simulink model "angle_lut_stage4_harness"  (R2024b)
settings: Solver=VariableStepAuto  StartTime=0.0  StopTime=10.0  RelTol=1e-3
model workspace (MAT data in the model file):
  B = 0.008
  BW_I = 5000
  BW_speed = 20
  J = 5.5e-06
  Ld = 6.1e-05
  Lq = 6.1e-05
  Rs = 0.09
  T_ident = 5e-05
  Ts = 5e-06
  Vdc = 24
  adc_current_bits = 12
  adc_current_gain = 1
  adc_current_lsb_A = 0.02442002442
  adc_current_noise_hz = 137
  adc_current_noise_std_A = 0.005
  adc_current_offset_a_A = 0
  adc_current_offset_b_A = 0
  adc_current_offset_c_A = 0
  adc_current_range_A = 50
  angle_sample_period_s = 5e-05
  encoder_counts_per_rev = 1024
  encoder_error_amp1_m_rad = 0.010471975512
  encoder_error_amp2_m_rad = 0.00523598775598
  encoder_error_bias_m_rad = 0
  encoder_error_mode = 2
  encoder_error_phase1_rad = 0
  encoder_error_phase2_rad = 0.785398163397
  encoder_noise_hz = 83
  encoder_noise_seed = 20260818
  encoder_noise_std_m_rad = 0
  encoder_speed_lsb_radps = 0.001
  encoder_speed_noise_hz = 41
  encoder_speed_noise_radps = 0.001
  encoder_speed_offset_radps = 0
  encoder_theta_noise_rad = 0.0001
  encoder_theta_offset_rad = 0
  fpwm = 20000
  inverter_voltage_drop_V = 0
  pn = 21
  psif = 0.004208
  pwm_deadtime_s = 0
  pwm_max_duty = 1
  pwm_min_duty = 0
  pwm_min_pulse_duty = 0
  sensor_mode = 1
  stage1_current_noise_seed = 20260818
  stage1_current_noise_std_A = 0
  stage1_ident_phase_s = 5e-06
  stage1_idq_initial_A = [0 0]
  stage1_load_torque_Nm = 0
  stage1_omega_m_initial_radps = 0
  stage1_overmod_epsilon = 1e-12
  stage1_speed_initial_revps = 0
  stage1_speed_pi_initial_A = 0
  stage1_speed_target_rpm = 1.59154943092
  stage2_active_enable = 0
  stage2_runtime_lut_e_rad = [0 0 0 0 0 0 0 0 0 0 0 0 ... (512 elements, 512x1)]
  stage2_runtime_nodes = 512
  stage3_active_enable = 0
  stage3_runtime_lut_e_rad = [0 0 0 0 0 0 0 0 0 0 0 0 ... (512 elements, 512x1)]
  stage3_runtime_nodes = 512
  stage4_active_enable = 0
  stage4_runtime_lut_e_rad = [0 0 0 0 0 0 0 0 0 0 0 0 ... (512 elements, 512x1)]
  stage4_runtime_nodes = 512
  theta0_e_rad = 0
undefined symbols (not defined in the file or in its folder): DiscIntNeverNeededParam
libraries: slpidlib x4, simulink x3, mcbplantlib x1, autolibpmsmexterior x1, spspowerguiLib x1
(part 2 of 2)

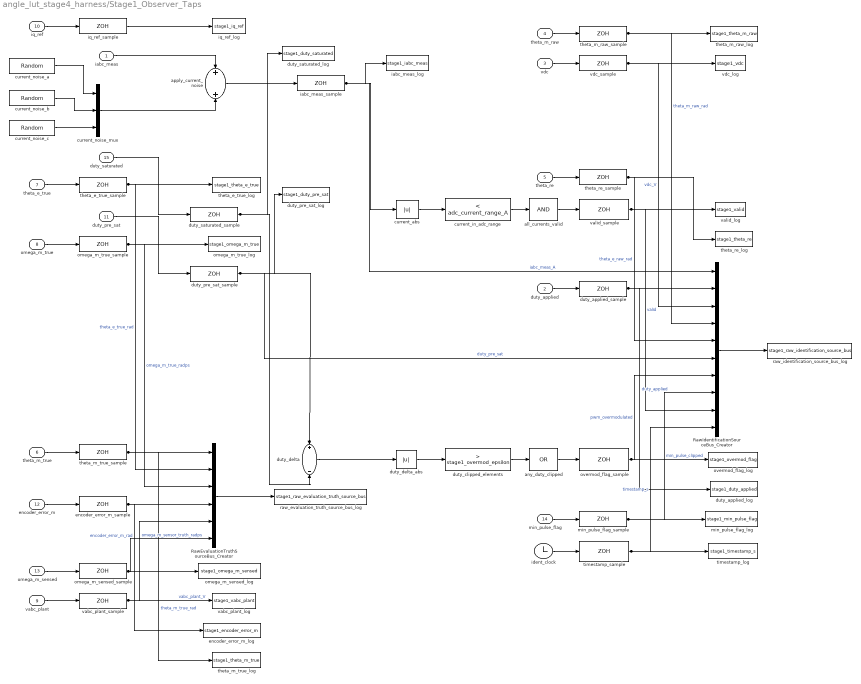
== system angle_lut_stage4_harness/Stage1_Observer_Taps ==
  iabc_meas : Inport
  duty_applied : Inport  Port=2
  vdc : Inport  Port=3
  theta_m_raw : Inport  Port=4
  theta_re : Inport  Port=5
  theta_m_true : Inport  Port=6
  theta_e_true : Inport  Port=7
  omega_m_true : Inport  Port=8
  vabc_plant : Inport  Port=9
  iq_ref : Inport  Port=10
  duty_pre_sat : Inport  Port=11
  encoder_error_m : Inport  Port=12
  omega_m_sensed : Inport  Port=13
  min_pulse_flag : Inport  Port=14
  duty_saturated : Inport  Port=15
  RawEvaluationTruthSourceBus_Creator : BusCreator  Inputs=6
  RawIdentificationSourceBus_Creator : BusCreator  Inputs=10
  all_currents_valid : Logic  Inputs=1  AllPortsSameDT=off  OutDataTypeStr=boolean
  any_duty_clipped : Logic  Operator=OR  Inputs=1  AllPortsSameDT=off  OutDataTypeStr=boolean
  apply_current_noise : Sum
  current_abs : Abs  SaturateOnIntegerOverflow=off
  current_in_adc_range : simulink/Logic and Bit Operations/Compare To Constant  relop=<  const=adc_current_range_A  OutDataTypeStr=boolean
  current_noise_a : RandomNumber  Variance=stage1_current_noise_std_A^2  Seed=double(stage1_current_noise_seed)  SampleTime=T_ident
  current_noise_b : RandomNumber  Variance=stage1_current_noise_std_A^2  Seed=double(stage1_current_noise_seed)+1  SampleTime=T_ident
  current_noise_c : RandomNumber  Variance=stage1_current_noise_std_A^2  Seed=double(stage1_current_noise_seed)+2  SampleTime=T_ident
  current_noise_mux : Mux  Inputs=3
  duty_applied_log : ToWorkspace  VariableName=stage1_duty_applied  SaveFormat=Timeseries  SampleTime=-1
  duty_applied_sample : ZeroOrderHold  SampleTime=[T_ident stage1_ident_phase_s]
  duty_clipped_elements : simulink/Logic and Bit Operations/Compare To Constant  relop=>  const=stage1_overmod_epsilon  OutDataTypeStr=boolean
  duty_delta : Sum  Inputs=+-
  duty_delta_abs : Abs  SaturateOnIntegerOverflow=off
  duty_pre_sat_log : ToWorkspace  VariableName=stage1_duty_pre_sat  SaveFormat=Timeseries  SampleTime=-1
  duty_pre_sat_sample : ZeroOrderHold  SampleTime=[T_ident stage1_ident_phase_s]
  duty_saturated_log : ToWorkspace  VariableName=stage1_duty_saturated  SaveFormat=Timeseries  SampleTime=-1
  duty_saturated_sample : ZeroOrderHold  SampleTime=[T_ident stage1_ident_phase_s]
  encoder_error_m_log : ToWorkspace  VariableName=stage1_encoder_error_m  SaveFormat=Timeseries  SampleTime=-1
  encoder_error_m_sample : ZeroOrderHold  SampleTime=[T_ident stage1_ident_phase_s]
  iabc_meas_log : ToWorkspace  VariableName=stage1_iabc_meas  SaveFormat=Timeseries  SampleTime=-1
  iabc_meas_sample : ZeroOrderHold  SampleTime=[T_ident stage1_ident_phase_s]
  ident_clock : Clock
  iq_ref_log : ToWorkspace  VariableName=stage1_iq_ref  SaveFormat=Timeseries  SampleTime=-1
  iq_ref_sample : ZeroOrderHold  SampleTime=[T_ident stage1_ident_phase_s]
  min_pulse_flag_log : ToWorkspace  VariableName=stage1_min_pulse_flag  SaveFormat=Timeseries  SampleTime=-1
  min_pulse_flag_sample : ZeroOrderHold  SampleTime=[T_ident stage1_ident_phase_s]
  omega_m_sensed_log : ToWorkspace  VariableName=stage1_omega_m_sensed  SaveFormat=Timeseries  SampleTime=-1
  omega_m_sensed_sample : ZeroOrderHold  SampleTime=[T_ident stage1_ident_phase_s]
  omega_m_true_log : ToWorkspace  VariableName=stage1_omega_m_true  SaveFormat=Timeseries  SampleTime=-1
  omega_m_true_sample : ZeroOrderHold  SampleTime=[T_ident stage1_ident_phase_s]
  overmod_flag_log : ToWorkspace  VariableName=stage1_overmod_flag  SaveFormat=Timeseries  SampleTime=-1
  overmod_flag_sample : ZeroOrderHold  SampleTime=[T_ident stage1_ident_phase_s]
  raw_evaluation_truth_source_bus_log : ToWorkspace  VariableName=stage1_raw_evaluation_truth_source_bus  SaveFormat=Timeseries  SampleTime=-1
  raw_identification_source_bus_log : ToWorkspace  VariableName=stage1_raw_identification_source_bus  SaveFormat=Timeseries  SampleTime=-1
  theta_e_true_log : ToWorkspace  VariableName=stage1_theta_e_true  SaveFormat=Timeseries  SampleTime=-1
  theta_e_true_sample : ZeroOrderHold  SampleTime=[T_ident stage1_ident_phase_s]
  theta_m_raw_log : ToWorkspace  VariableName=stage1_theta_m_raw  SaveFormat=Timeseries  SampleTime=-1
  theta_m_raw_sample : ZeroOrderHold  SampleTime=[T_ident stage1_ident_phase_s]
  theta_m_true_log : ToWorkspace  VariableName=stage1_theta_m_true  SaveFormat=Timeseries  SampleTime=-1
  theta_m_true_sample : ZeroOrderHold  SampleTime=[T_ident stage1_ident_phase_s]
  theta_re_log : ToWorkspace  VariableName=stage1_theta_re  SaveFormat=Timeseries  SampleTime=-1
  theta_re_sample : ZeroOrderHold  SampleTime=[T_ident stage1_ident_phase_s]
  timestamp_log : ToWorkspace  VariableName=stage1_timestamp_s  SaveFormat=Timeseries  SampleTime=-1
  timestamp_sample : ZeroOrderHold  SampleTime=[T_ident stage1_ident_phase_s]
  vabc_plant_log : ToWorkspace  VariableName=stage1_vabc_plant  SaveFormat=Timeseries  SampleTime=-1
  vabc_plant_sample : ZeroOrderHold  SampleTime=[T_ident stage1_ident_phase_s]
  valid_log : ToWorkspace  VariableName=stage1_valid  SaveFormat=Timeseries  SampleTime=-1
  valid_sample : ZeroOrderHold  SampleTime=[T_ident stage1_ident_phase_s]
  vdc_log : ToWorkspace  VariableName=stage1_vdc  SaveFormat=Timeseries  SampleTime=-1
  vdc_sample : ZeroOrderHold  SampleTime=[T_ident stage1_ident_phase_s]
  wires:
  theta_e_true/1 -> theta_e_true_sample/1
  current_abs/1 -> current_in_adc_range/1
  iq_ref/1 -> iq_ref_sample/1
  current_noise_a/1 -> current_noise_mux/1
  encoder_error_m/1 -> encoder_error_m_sample/1
  current_noise_b/1 -> current_noise_mux/2
  current_noise_c/1 -> current_noise_mux/3
  omega_m_true/1 -> omega_m_true_sample/1
  overmod_flag_sample/1 -> overmod_flag_log/1, RawIdentificationSourceBus_Creator/7  "pwm_overmodulated"
  theta_m_true/1 -> theta_m_true_sample/1
  omega_m_sensed/1 -> omega_m_sensed_sample/1
  valid_sample/1 -> valid_log/1, RawIdentificationSourceBus_Creator/9  "valid"
  vdc_sample/1 -> vdc_log/1, RawIdentificationSourceBus_Creator/3  "vdc_V"
  all_currents_valid/1 -> valid_sample/1
  vabc_plant/1 -> vabc_plant_sample/1
  iq_ref_sample/1 -> iq_ref_log/1
  omega_m_sensed_sample/1 -> omega_m_sensed_log/1, RawEvaluationTruthSourceBus_Creator/6  "omega_m_sensor_truth_radps"
  iabc_meas/1 -> apply_current_noise/1
  current_noise_mux/1 -> apply_current_noise/2
  duty_saturated/1 -> duty_saturated_sample/1
  theta_e_true_sample/1 -> theta_e_true_log/1, RawEvaluationTruthSourceBus_Creator/2  "theta_e_true_rad"
  duty_pre_sat/1 -> duty_pre_sat_sample/1
  vdc/1 -> vdc_sample/1
  RawEvaluationTruthSourceBus_Creator/1 -> raw_evaluation_truth_source_bus_log/1
  omega_m_true_sample/1 -> omega_m_true_log/1, RawEvaluationTruthSourceBus_Creator/3  "omega_m_true_radps"
  theta_m_true_sample/1 -> theta_m_true_log/1, RawEvaluationTruthSourceBus_Creator/1  "theta_m_true_rad"
  encoder_error_m_sample/1 -> encoder_error_m_log/1, RawEvaluationTruthSourceBus_Creator/4  "encoder_error_m_rad"
  duty_applied/1 -> duty_applied_sample/1
  vabc_plant_sample/1 -> vabc_plant_log/1, RawEvaluationTruthSourceBus_Creator/5  "vabc_plant_V"
  apply_current_noise/1 -> iabc_meas_sample/1
  duty_saturated_sample/1 -> duty_delta/2, duty_saturated_log/1
  duty_pre_sat_sample/1 -> duty_delta/1, duty_pre_sat_log/1, RawIdentificationSourceBus_Creator/6  "duty_pre_sat"
  iabc_meas_sample/1 -> iabc_meas_log/1, current_abs/1, RawIdentificationSourceBus_Creator/1  "iabc_meas_A"
  duty_delta/1 -> duty_delta_abs/1
  duty_delta_abs/1 -> duty_clipped_elements/1
  duty_applied_sample/1 -> RawIdentificationSourceBus_Creator/2, duty_applied_log/1  "duty_applied"
  current_in_adc_range/1 -> all_currents_valid/1
  min_pulse_flag/1 -> min_pulse_flag_sample/1
  duty_clipped_elements/1 -> any_duty_clipped/1
  theta_m_raw/1 -> theta_m_raw_sample/1
  theta_re/1 -> theta_re_sample/1
  any_duty_clipped/1 -> overmod_flag_sample/1
  ident_clock/1 -> timestamp_sample/1
  theta_m_raw_sample/1 -> theta_m_raw_log/1, RawIdentificationSourceBus_Creator/4  "theta_m_raw_rad"
  theta_re_sample/1 -> theta_re_log/1, RawIdentificationSourceBus_Creator/5  "theta_e_raw_rad"
  min_pulse_flag_sample/1 -> min_pulse_flag_log/1, RawIdentificationSourceBus_Creator/8  "min_pulse_clipped"
  timestamp_sample/1 -> timestamp_log/1, RawIdentificationSourceBus_Creator/10  "timestamp_s"
  RawIdentificationSourceBus_Creator/1 -> raw_identification_source_bus_log/1

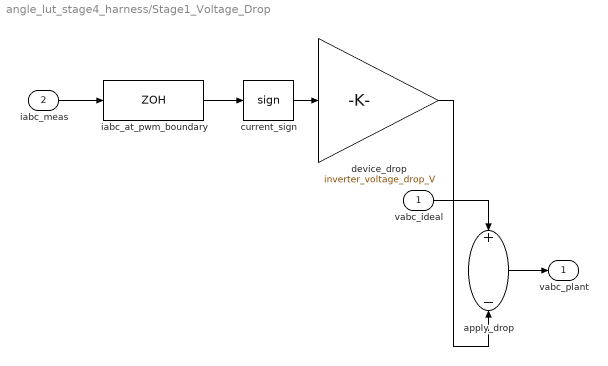
== system angle_lut_stage4_harness/Stage1_Voltage_Drop ==
  vabc_ideal : Inport
  iabc_meas : Inport  Port=2
  apply_drop : Sum  Inputs=+-
  current_sign : Signum
  device_drop : Gain  Gain=inverter_voltage_drop_V
  iabc_at_pwm_boundary : ZeroOrderHold  SampleTime=[T_ident 0]
  vabc_plant : Outport
  wires:
  iabc_meas/1 -> iabc_at_pwm_boundary/1
  current_sign/1 -> device_drop/1
  iabc_at_pwm_boundary/1 -> current_sign/1
  vabc_ideal/1 -> apply_drop/1
  device_drop/1 -> apply_drop/2
  apply_drop/1 -> vabc_plant/1

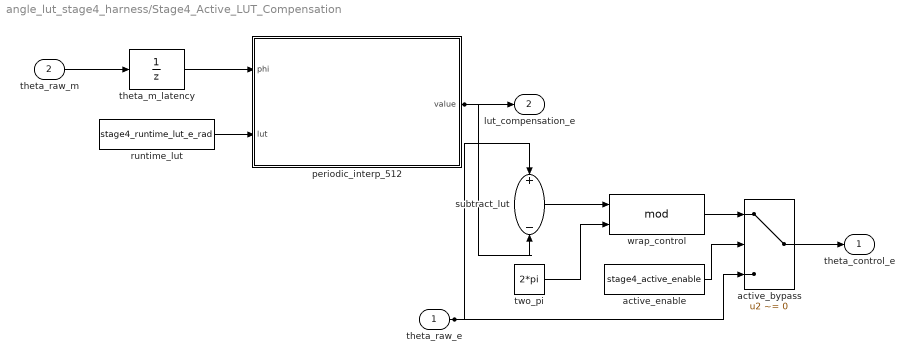
== system angle_lut_stage4_harness/Stage4_Active_LUT_Compensation ==
  theta_raw_e : Inport
  theta_raw_m : Inport  Port=2
  active_bypass : Switch  Criteria=u2 ~= 0  Threshold=0.5  SaturateOnIntegerOverflow=off  InputSameDT=off
  active_enable : Constant  Value=stage4_active_enable  OutDataTypeStr=boolean
  periodic_interp_512 : MATLAB Function  TreatAsAtomicUnit=on
  runtime_lut : Constant  Value=stage4_runtime_lut_e_rad
  subtract_lut : Sum  Inputs=+-
  theta_m_latency : UnitDelay  SampleTime=Ts  HasFrameUpgradeWarning=on
  two_pi : Constant  Value=2*pi
  wrap_control : Math  Operator=mod
  theta_control_e : Outport
  lut_compensation_e : Outport  Port=2
  wires:
  theta_raw_m/1 -> theta_m_latency/1
  theta_m_latency/1 -> periodic_interp_512/1(phi)
  two_pi/1 -> wrap_control/2
  runtime_lut/1 -> periodic_interp_512/2(lut)
  periodic_interp_512/1(value) -> subtract_lut/2, lut_compensation_e/1
  theta_raw_e/1 -> active_bypass/3, subtract_lut/1
  subtract_lut/1 -> wrap_control/1
  wrap_control/1 -> active_bypass/1
  active_enable/1 -> active_bypass/2
  active_bypass/1 -> theta_control_e/1

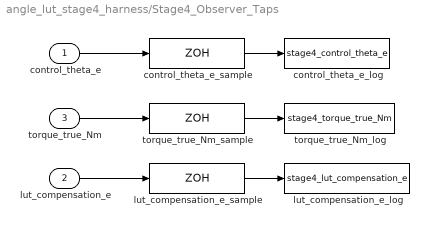
== system angle_lut_stage4_harness/Stage4_Observer_Taps ==
  control_theta_e : Inport
  lut_compensation_e : Inport  Port=2
  torque_true_Nm : Inport  Port=3
  control_theta_e_log : ToWorkspace  VariableName=stage4_control_theta_e  SaveFormat=Timeseries  SampleTime=-1
  control_theta_e_sample : ZeroOrderHold  SampleTime=[T_ident stage1_ident_phase_s]
  lut_compensation_e_log : ToWorkspace  VariableName=stage4_lut_compensation_e  SaveFormat=Timeseries  SampleTime=-1
  lut_compensation_e_sample : ZeroOrderHold  SampleTime=[T_ident stage1_ident_phase_s]
  torque_true_Nm_log : ToWorkspace  VariableName=stage4_torque_true_Nm  SaveFormat=Timeseries  SampleTime=-1
  torque_true_Nm_sample : ZeroOrderHold  SampleTime=[T_ident stage1_ident_phase_s]
  wires:
  control_theta_e/1 -> control_theta_e_sample/1
  torque_true_Nm_sample/1 -> torque_true_Nm_log/1
  torque_true_Nm/1 -> torque_true_Nm_sample/1
  lut_compensation_e_sample/1 -> lut_compensation_e_log/1
  control_theta_e_sample/1 -> control_theta_e_log/1
  lut_compensation_e/1 -> lut_compensation_e_sample/1

== matlab function angle_lut_stage4_harness/MATLAB Function9 ==
  data: Iq input; s output; We input; Lq input
function s = F1(Iq,We,Lq)
    %Lq=0.3;

    s=Iq*We*Lq;

== matlab function angle_lut_stage4_harness/MATLAB Function10 ==
  data: Id input; s output; We input; Ld input; flux input
function s = F2(Id,We,Ld,flux)
    %Ld=0.15;
    %flux=3;

    s=We*(Ld*Id+flux);

== matlab function angle_lut_stage4_harness/Stage1_Duty_Nonideal/Apply_Duty_Nonidealities ==
  data: duty_cmd input; duty_eff output; iabc input; min_pulse input; deadtime_s input; ident_period_s input; duty_min input; duty_max input; min_pulse_flag output
function [duty_eff,min_pulse_flag] = f(duty_cmd,iabc,min_pulse,deadtime_s,ident_period_s,duty_min,duty_max)
duty_eff = duty_cmd;
min_pulse_flag = false;
for k = 1:3
    d = duty_cmd(k);
    if (d > duty_min) && (d < duty_min + min_pulse)
        duty_eff(k) = duty_min;
        min_pulse_flag = true;
    elseif (d < duty_max) && (d > duty_max - min_pulse)
        duty_eff(k) = duty_max;
        min_pulse_flag = true;
    end
end
dead_fraction = deadtime_s / ident_period_s;
for k = 1:3
    duty_eff(k) = duty_eff(k) - dead_fraction*sign(iabc(k));
    duty_eff(k) = min(max(duty_eff(k),duty_min),duty_max);
end
end

== matlab function angle_lut_stage4_harness/MATLAB Function3 ==
  data: Ialpha output; Ia input; Ib input; Ic input; Ibeta output
function[Ialpha,Ibeta]=  CLARK(Ia,Ib,Ic)
    



    Ialpha=2/3*(Ia-Ib/2-Ic/2);
    Ibeta=2/3*(Ib*sqrt(3)/2-Ic*sqrt(3)/2);

== matlab function angle_lut_stage4_harness/MATLAB Function2 ==
  data: CMPA output; m input; sector input; theta input; CMPB output; CMPC output; Tpwm input
function[CMPA,CMPB,CMPC]=  SVPWM(m,sector,theta,Tpwm)
    



    CMPA=0;
    CMPB=0;
    CMPC=0;



%T0和Tpwm为PWM周期，实际会被消除掉（三角波调制部分，进行归一化）
    T0=Tpwm;

%m表示为调制深度/直流电压利用率
if m<0
    m=-m;
    sector=sector+3;
    sector=mod(sector,6);
end

%计算工作时间
    tx=m*T0*sin(pi/3-theta);
    ty=m*T0*sin(theta);
    t0=T0-tx-ty;

    if (t0 < 0)
        Tsum = tx + ty;
        tx = tx/Tsum*T0;
        ty = ty/Tsum*T0;
        t0 = 0;
    end

switch sector
   case 2
        th = tx;
        tx = ty;
        ty = th;
   case 4
        th = tx;
        tx = ty;
        ty = th;
   case 6
        th = tx;
        tx = ty;
        ty = th;
   otherwise 
          
end

    
    CL=t0/2/T0;
    CM=CL+tx/T0;
    CH=CM+ty/T0;


    switch sector
    case 1
        CMPA = CL;
        CMPB = CM;
        CMPC = CH;
    case 2
        CMPA = CM;
        CMPB = CL;
        CMPC = CH;
    case 3
        CMPA = CH;
        CMPB = CL;
        CMPC = CM;
    case 4
        CMPA = CH;
        CMPB = CM;
        CMPC = CL;
    case 5
        CMPA = CM;
        CMPB = CH;
        CMPC = CL;
    case 6
        CMPA = CL;
        CMPB = CH;
        CMPC = CM;
    otherwise 
        CMPA = CL;  % 不会进入这个分支
        CMPB = CH;
        CMPC = CM;    
    end

    CMPA = 1- CMPA;
    CMPB = 1- CMPB;
    CMPC = 1- CMPC;

== matlab function angle_lut_stage4_harness/MATLAB Function4 ==
  data: Iq output; Ialpha input; Ibeta input; Id output; theta input
function[Iq,Id]=  PARK(Ialpha,Ibeta,theta)


%theta=-theta;

Id =  Ialpha*cos(theta) + Ibeta*sin(theta);
Iq = -Ialpha*sin(theta) + Ibeta*cos(theta);

== matlab function angle_lut_stage4_harness/MATLAB Function5 ==
  data: Valpha output; Vq input; Vd input; Vbeta output; theta input
function[Valpha,Vbeta]=  ANTIPARK(Vq,Vd,theta)


%theta=-theta;


Valpha=Vd*cos(theta) - Vq*sin(theta);
Vbeta=Vd*sin(theta) + Vq*cos(theta);

== matlab function angle_lut_stage4_harness/Stage4_Active_LUT_Compensation/periodic_interp_512 ==
  data: phi input; value output; lut input
function value = f(phi,lut)
%#codegen
M = 512;
phi = mod(phi,2*pi);
u = M*phi/(2*pi);
j0z = floor(u);
alpha = u-j0z;
j0 = j0z+1;
j1 = mod(j0z+1,M)+1;
value = (1-alpha)*lut(j0)+alpha*lut(j1);
end

== matlab function angle_lut_stage4_harness/MATLAB Function7 ==
  data: m output; Valpha input; Vbeta input; sector output; theta output
function[m,sector,theta]= cal_para(Valpha,Vbeta)

    Va =  Valpha;
    Vb = -0.5*Valpha + sqrt(3)/2*Vbeta;
    Vc = -0.5*Valpha - sqrt(3)/2*Vbeta;
    
   
    if Valpha==0 && Vbeta > 0
        theta = 90;
    elseif Valpha==0 && Vbeta < 0
        theta = 270;
    elseif Valpha > 0 && Vbeta >= 0
        theta = atan(Vbeta/Valpha)/(2*pi)*360;
    elseif Valpha > 0 && Vbeta <= 0
        theta = atan(Vbeta/Valpha)/(2*pi)*360+360;
    elseif Valpha < 0 && Vbeta >= 0
        theta = atan(Vbeta/Valpha)/(2*pi)*360+180;
    elseif Valpha < 0 && Vbeta <= 0
        theta = atan(Vbeta/Valpha)/(2*pi)*360+180;
    else
        theta = 0;
    end
    
    %angle2=theta;
    if Vbeta~=0
        angle2=Vbeta/Valpha;
    else
        angle2 =0;
    end
    angle= theta;

     % 判断所属的扇区
    if angle >= 0 && angle < 60
        sector = 1;
        theta = angle;
    elseif angle >= 60 && angle < 120
        sector = 2;
        theta = angle - 60;
    elseif angle >= 120 && angle < 180
        sector = 3;
        theta = angle - 120;
    elseif angle >= 180 && angle < 240
        sector = 4;
        theta = angle - 180;
    elseif angle >= 240 && angle < 300
        sector = 5;
        theta = angle - 240;
    else
        sector = 6;
        theta = angle - 300;
    end
    
    Vout=sqrt(Valpha*Valpha+Vbeta*Vbeta);
    m=Vout/sqrt(3)*2;

%theta=-theta;
